simulink model "compwithsimply27"  (R2021a)
settings: Solver=VariableStepAuto  StartTime=0.0  StopTime=10.0  RelTol=1e-3
undefined symbols (not defined in the file): Newton, Raphson
settings Model: Creator=CMelt  LastModifiedBy=CMelt

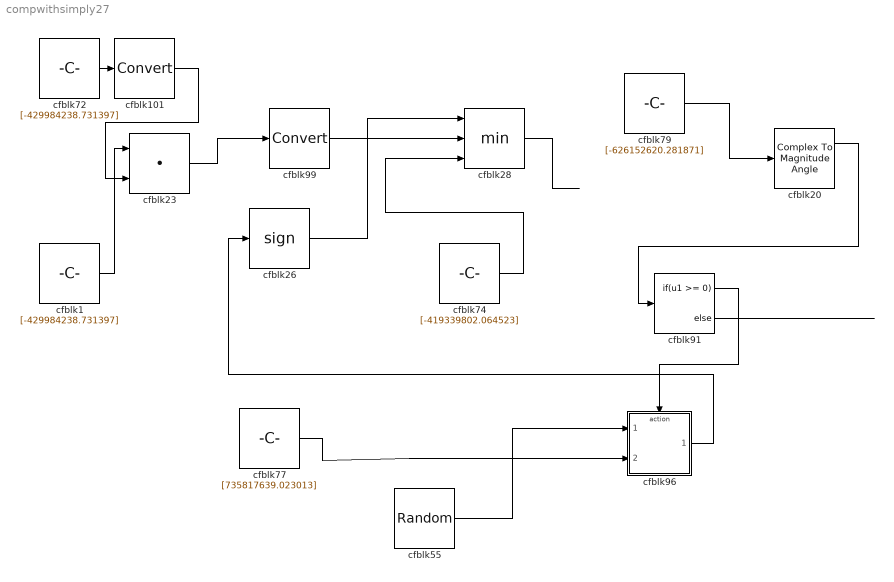
== system compwithsimply27 ==
  cfblk1 : Constant  Value=[-429984238.731397]  SampleTime=1
  cfblk101 : DataTypeConversion
  cfblk20 : ComplexToMagnitudeAngle
  cfblk23 : DotProduct  InputSameDT=on  OutDataTypeStr=Inherit: Inherit via internal rule
  cfblk26 : Signum
  cfblk28 : MinMax  Inputs=3
  cfblk55 : RandomNumber  Mean=[-1249.450853]  Variance=[75448.037597]  Seed=[754077994.000000]  SampleTime=0.1
  cfblk72 : Constant  Value=[-429984238.731397]  SampleTime=1
  cfblk74 : Constant  Value=[-419339802.064523]  SampleTime=1
  cfblk77 : Constant  Value=[735817639.023013]  SampleTime=1
  cfblk79 : Constant  Value=[-626152620.281871]  SampleTime=1
  cfblk91 : If  IfExpression=u1 >= 0  SampleTime=1
  cfblk96 : Subsystem  TreatAsAtomicUnit=on
  cfblk99 : DataTypeConversion
  wires:
  cfblk26/1 -> cfblk28/1
  cfblk96/1(cfblk2) -> cfblk26/1
  cfblk77/1 -> cfblk96/2(cfblk7)
  cfblk55/1 -> cfblk96/1(cfblk1)
  cfblk99/1 -> cfblk28/2
  cfblk23/1 -> cfblk99/1
  cfblk101/1 -> cfblk23/2
  cfblk74/1 -> cfblk28/3
  cfblk72/1 -> cfblk101/1
  cfblk1/1 -> cfblk23/1
  cfblk91/1 -> cfblk96/Action
  cfblk79/1 -> cfblk20/1
  cfblk20/1 -> cfblk91/1
  cfblk28/1 -> ?
  cfblk91/2 -> ?

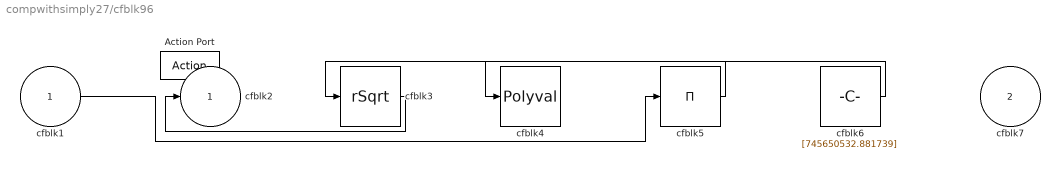
== system compwithsimply27/cfblk96 ==
  cfblk1 : Inport
  cfblk7 : Inport  Port=2
  Action Port : ActionPort  ActionPortLabel=if(u1 >= 0)
  cfblk3 : Sqrt  Operator=rSqrt  AlgorithmType=Newton-Raphson  SaturateOnIntegerOverflow=on
  cfblk4 : Polyval  Coefs=[ +2.081618890e-019, -1.441693666e-014, +4.719686976e-010, -8.536869453e-006, +1.621573104e-001, -8.087801117e+001 ]
  cfblk5 : Product  Inputs=*
  cfblk6 : Constant  Value=[745650532.881739]  SampleTime=1
  cfblk2 : Outport
  wires:
  cfblk3/1 -> cfblk2/1
  cfblk6/1 -> cfblk4/1
  cfblk1/1 -> cfblk5/1
  cfblk5/1 -> cfblk3/1
